simulink model "send_nad_r2018b"  (R2018b)
settings: Solver=VariableStepAuto  StartTime=0.0  StopTime=10.0  RelTol=1e-3
libraries: lib_ed247 x2
settings Model: EnablePacing=on  Creator=odufour  LastModifiedBy=odufour
settings DataIOCC: ExternalInput=ds  ReturnWorkspaceOutputs=on

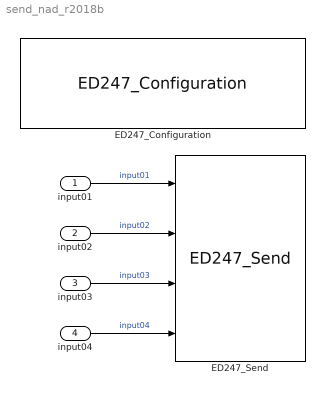
== system send_nad_r2018b ==
  input01 : Inport  OutDataTypeStr=uint8  SampleTime=0.5
  input02 : Inport  Port=2  OutDataTypeStr=uint8  SampleTime=0.5
  input03 : Inport  Port=3  OutDataTypeStr=uint8  SampleTime=0.5
  input04 : Inport  Port=4  OutDataTypeStr=single  PortDimensions=[2,2]  SampleTime=0.5
  ED247_Configuration : lib_ed247/ED247_Configuration  configurationFilename='ecic_func_exchange_nad_uc_main.xml'  enableLog=off  logFilename=''
      settings: SourceProductName=Airbus ED247
  ED247_Send : lib_ed247/ED247_Send  SFunctionModules=''
      settings: SourceProductName=Airbus ED247
  wires:
  input01/1 -> ED247_Send/1  "input01"
  input02/1 -> ED247_Send/2  "input02"
  input03/1 -> ED247_Send/3  "input03"
  input04/1 -> ED247_Send/4  "input04"
